simulink model "MyPTControl_RTW"  (R2022a)
settings: Solver=ode1  StartTime=0.0  StopTime=inf  FixedStep=0.001  RelTol=1e-3
PreLoadFcn:
  | vehicle = 'Car'; if ~length(which('cmself')), cmenv; end
  | MyPTControl_RTW_bus
InitFcn:
  | vehicle = 'Car'; if ~length(which('cmself')), cmenv; end
  | MyPTControl_RTW_bus
undefined symbols (not defined in the file or in its folder): EngineOut_Load, EngineOut_set_ISC, Ignition, ISGOut_Load, OperationState
libraries: simulink x11
(part 1 of 2)
Description:
  | CarMaker Plug-in Model Target
settings Model: ModifiedByFormat=IPG  Creator=ml  LastModifiedBy=IPG
settings DebuggingCC: UnconnectedInputMsg=warning  UnconnectedOutputMsg=warning  UnconnectedLineMsg=warning
settings RTWCC: Description=CarMaker Plug-in Model Target  SystemTargetFile=CarMaker.tlc  TemplateMakefile=CarMaker_unix-win64.tmf  DLArmComputeVersion=19.05
settings CodeAppCC: MaxIdLength=127
settings STFCustomTargetCC: TargetLangStandard=C99 (ISO)  CombineOutputUpdateFcns=on  MatFileLogging=on  CodeInterfacePackaging=Reusable function  GRTInterface=off  GenerateAllocFcn=on  SystemTargetFile=CarMaker.tlc
settings GRTTargetCC: ParMdlRefBuildCompliant=off  CompOptLevelCompliant=off  ConcurrentExecutionCompliant=off  CodeInterfacePackaging=Reusable function  CPPClassGenCompliant=off  GenerateAllocFcn=on  UseToolchainInfoCompliant=off

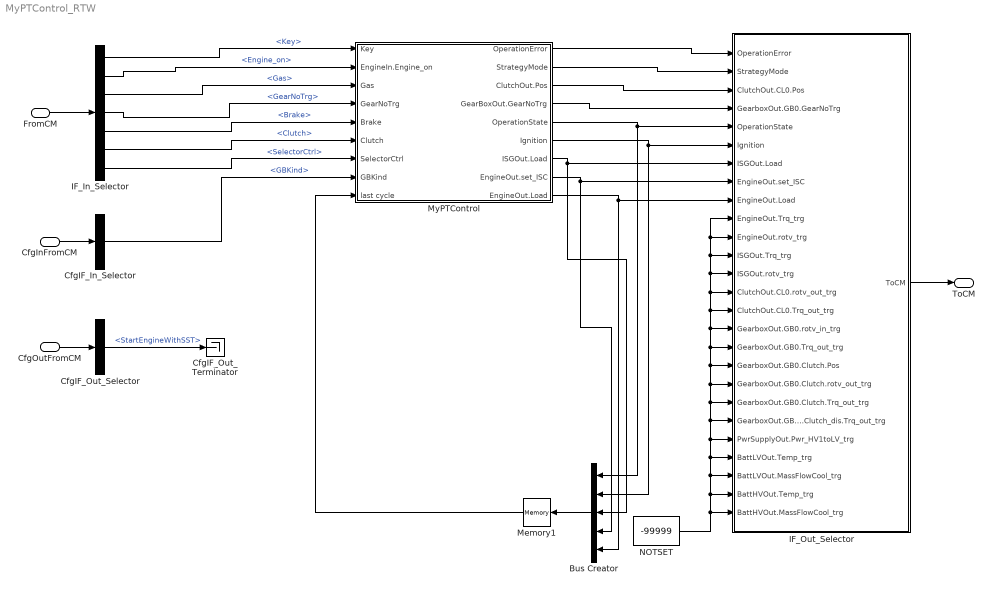
== system MyPTControl_RTW ==
  FromCM : Inport  OutDataTypeStr=Bus: cmPTControlIn
  CfgInFromCM : Inport  Port=2  OutDataTypeStr=Bus: cmPTControlCfgIn
  CfgOutFromCM : Inport  Port=3  OutDataTypeStr=Bus: cmPTControlCfgOut
  Bus Creator : BusCreator  Inputs=5
  CfgIF_In_Selector : BusSelector  OutputSignals=Gearbox.GB0.GBKind
  CfgIF_Out_Selector : BusSelector  OutputSignals=StartEngineWithSST
  CfgIF_Out_Terminator : Terminator
  IF_In_Selector : BusSelector  OutputSignals=Key,EngineIn.Engine_on,Gas,GearNoTrg,Brake,Clutch,SelectorCtrl
  IF_Out_Selector : Subsystem  mask(Signal Selection){}
      mask help: Signal Selection Block
      settings: OpenFcn=cmSignalSelect('SignalSelection_CB',gcb)
  Memory1 : Memory
  MyPTControl : Subsystem
  NOTSET : Constant  Value=-99999
  ToCM : Outport  OutDataTypeStr=Bus: cmPTControlOut
  wires:
  FromCM/1 -> IF_In_Selector/1
  IF_Out_Selector/1(ToCM) -> ToCM/1
  CfgInFromCM/1 -> CfgIF_In_Selector/1
  CfgOutFromCM/1 -> CfgIF_Out_Selector/1
  CfgIF_Out_Selector/1 -> CfgIF_Out_Terminator/1  "<StartEngineWithSST>"
  Bus Creator/1 -> Memory1/1
  MyPTControl/6(Ignition) -> IF_Out_Selector/6(Ignition), Bus Creator/2
  IF_In_Selector/2 -> MyPTControl/2(EngineIn.Engine_on)  "<Engine_on>"
  IF_In_Selector/6 -> MyPTControl/6(Clutch)  "<Clutch>"
  IF_In_Selector/3 -> MyPTControl/3(Gas)  "<Gas>"
  MyPTControl/1(OperationError) -> IF_Out_Selector/1(OperationError)
  CfgIF_In_Selector/1 -> MyPTControl/8(GBKind)  "<GBKind>"
  MyPTControl/4(GearBoxOut.GearNoTrg) -> IF_Out_Selector/4(GearboxOut.GB0.GearNoTrg)
  IF_In_Selector/4 -> MyPTControl/4(GearNoTrg)  "<GearNoTrg>"
  MyPTControl/7(ISGOut.Load) -> IF_Out_Selector/7(ISGOut.Load), Bus Creator/3
  IF_In_Selector/5 -> MyPTControl/5(Brake)  "<Brake>"
  MyPTControl/5(OperationState) -> IF_Out_Selector/5(OperationState), Bus Creator/1
  MyPTControl/8(EngineOut.set_ISC) -> IF_Out_Selector/8(EngineOut.set_ISC), Bus Creator/4
  IF_In_Selector/1 -> MyPTControl/1(Key)  "<Key>"
  MyPTControl/2(StrategyMode) -> IF_Out_Selector/2(StrategyMode)
  MyPTControl/3(ClutchOut.Pos) -> IF_Out_Selector/3(ClutchOut.CL0.Pos)
  Memory1/1 -> MyPTControl/9(last cycle)
  MyPTControl/9(EngineOut.Load) -> IF_Out_Selector/9(EngineOut.Load), Bus Creator/5
  NOTSET/1 -> IF_Out_Selector/26(BattHVOut.MassFlowCool_trg), IF_Out_Selector/25(BattHVOut.Temp_trg), IF_Out_Selector/24(BattLVOut.MassFlowCool_trg), IF_Out_Selector/23(BattLVOut.Temp_trg), IF_Out_Selector/22(PwrSupplyOut.Pwr_HV1toLV_trg), IF_Out_Selector/21(GearboxOut.GB0.Clutch_dis.Trq_out_trg), IF_Out_Selector/20(GearboxOut.GB0.Clutch.Trq_out_trg), IF_Out_Selector/19(GearboxOut.GB0.Clutch.rotv_out_trg), IF_Out_Selector/18(GearboxOut.GB0.Clutch.Pos), IF_Out_Selector/17(GearboxOut.GB0.Trq_out_trg), IF_Out_Selector/16(GearboxOut.GB0.rotv_in_trg), IF_Out_Selector/15(ClutchOut.CL0.Trq_out_trg), IF_Out_Selector/14(ClutchOut.CL0.rotv_out_trg), IF_Out_Selector/13(ISGOut.rotv_trg), IF_Out_Selector/12(ISGOut.Trq_trg), IF_Out_Selector/10(EngineOut.Trq_trg), IF_Out_Selector/11(EngineOut.rotv_trg)
  IF_In_Selector/7 -> MyPTControl/7(SelectorCtrl)  "<SelectorCtrl>"

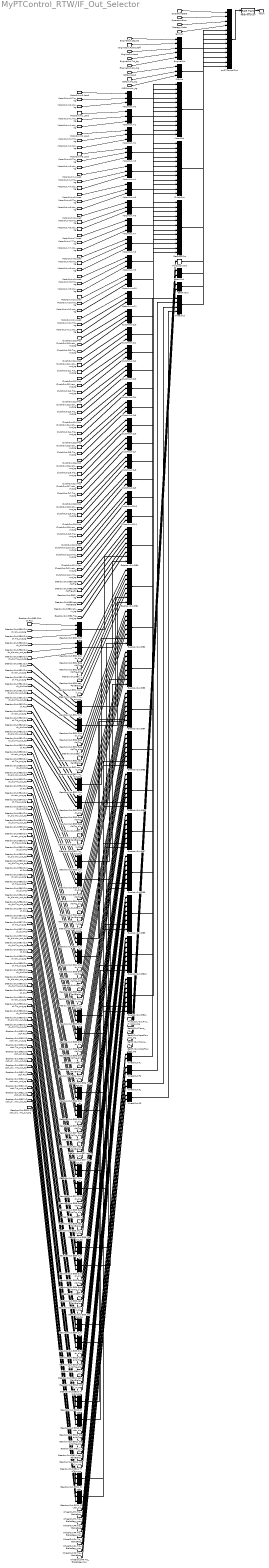
== system MyPTControl_RTW/IF_Out_Selector ==
  OperationError : Inport
  StrategyMode : Inport  Port=2
  ClutchOut.CL0.Pos : Inport  Port=3
  GearboxOut.GB0.GearNoTrg : Inport  Port=4
  OperationState : Inport  Port=5
  Ignition : Inport  Port=6
  ISGOut.Load : Inport  Port=7
  EngineOut.set_ISC : Inport  Port=8
  EngineOut.Load : Inport  Port=9
  EngineOut.Trq_trg : Inport  Port=10
  EngineOut.rotv_trg : Inport  Port=11
  ISGOut.Trq_trg : Inport  Port=12
  ISGOut.rotv_trg : Inport  Port=13
  ClutchOut.CL0.rotv_out_trg : Inport  Port=14
  ClutchOut.CL0.Trq_out_trg : Inport  Port=15
  GearboxOut.GB0.rotv_in_trg : Inport  Port=16
  GearboxOut.GB0.Trq_out_trg : Inport  Port=17
  GearboxOut.GB0.Clutch.Pos : Inport  Port=18
  GearboxOut.GB0.Clutch.rotv_out_trg : Inport  Port=19
  GearboxOut.GB0.Clutch.Trq_out_trg : Inport  Port=20
  GearboxOut.GB0.Clutch_dis.Trq_out_trg : Inport  Port=21
  PwrSupplyOut.Pwr_HV1toLV_trg : Inport  Port=22
  BattLVOut.Temp_trg : Inport  Port=23
  BattLVOut.MassFlowCool_trg : Inport  Port=24
  BattHVOut.Temp_trg : Inport  Port=25
  BattHVOut.MassFlowCool_trg : Inport  Port=26
  BattHVOut : BusCreator  Inputs=2
  BattLVOut : BusCreator  Inputs=2
  ClutchOut : BusCreator  Inputs=12
  ClutchOut.CL{0..11} (12 alike) : BusCreator  Inputs=3
  ClutchOut.CL1.Pos : Constant  Value=0
  ClutchOut.CL1.Trq_out_trg : Constant  Value=0
  ClutchOut.CL1.rotv_out_trg : Constant  Value=0
  ClutchOut.CL10.Pos : Constant  Value=0
  ClutchOut.CL10.Trq_out_trg : Constant  Value=0
  ClutchOut.CL10.rotv_out_trg : Constant  Value=0
  ClutchOut.CL11.Pos : Constant  Value=0
  ClutchOut.CL11.Trq_out_trg : Constant  Value=0
  ClutchOut.CL11.rotv_out_trg : Constant  Value=0
  ClutchOut.CL2.Pos : Constant  Value=0
  ClutchOut.CL2.Trq_out_trg : Constant  Value=0
  ClutchOut.CL2.rotv_out_trg : Constant  Value=0
  ClutchOut.CL3.Pos : Constant  Value=0
  ClutchOut.CL3.Trq_out_trg : Constant  Value=0
  ClutchOut.CL3.rotv_out_trg : Constant  Value=0
  ClutchOut.CL4.Pos : Constant  Value=0
  ClutchOut.CL4.Trq_out_trg : Constant  Value=0
  ClutchOut.CL4.rotv_out_trg : Constant  Value=0
  ClutchOut.CL5.Pos : Constant  Value=0
  ClutchOut.CL5.Trq_out_trg : Constant  Value=0
  ClutchOut.CL5.rotv_out_trg : Constant  Value=0
  ClutchOut.CL6.Pos : Constant  Value=0
  ClutchOut.CL6.Trq_out_trg : Constant  Value=0
  ClutchOut.CL6.rotv_out_trg : Constant  Value=0
  ClutchOut.CL7.Pos : Constant  Value=0
  ClutchOut.CL7.Trq_out_trg : Constant  Value=0
  ClutchOut.CL7.rotv_out_trg : Constant  Value=0
  ClutchOut.CL8.Pos : Constant  Value=0
  ClutchOut.CL8.Trq_out_trg : Constant  Value=0
  ClutchOut.CL8.rotv_out_trg : Constant  Value=0
  ClutchOut.CL9.Pos : Constant  Value=0
  ClutchOut.CL9.Trq_out_trg : Constant  Value=0
  ClutchOut.CL9.rotv_out_trg : Constant  Value=0
  EngineOut : BusCreator  Inputs=5
  EngineOut.FuelCutOff : Constant  Value=0
  GearboxOut : BusCreator  Inputs=12
  GearboxOut.GB{0..11} (12 alike) : BusCreator  Inputs=8
  GearboxOut.GB0.Clutch : BusCreator  Inputs=3
  GearboxOut.GB0.Clutch_dis : BusCreator  Inputs=3
  GearboxOut.GB0.Clutch_dis.Pos : Constant  Value=0
  GearboxOut.GB0.Clutch_dis.rotv_out_trg : Constant  Value=0
  GearboxOut.GB0.GearNoTrg_dis : Constant  Value=0
  GearboxOut.GB0.i_trg : Constant  Value=0
  GearboxOut.GB0.set_ParkBrake : Constant  Value=0
  GearboxOut.GB1.Clutch : BusCreator  Inputs=3
  GearboxOut.GB1.Clutch.Pos : Constant  Value=0
  GearboxOut.GB1.Clutch.Trq_out_trg : Constant  Value=0
  GearboxOut.GB1.Clutch.rotv_out_trg : Constant  Value=0
  GearboxOut.GB1.Clutch_dis : BusCreator  Inputs=3
  GearboxOut.GB1.Clutch_dis.Pos : Constant  Value=0
  GearboxOut.GB1.Clutch_dis.Trq_out_trg : Constant  Value=0
  GearboxOut.GB1.Clutch_dis.rotv_out_trg : Constant  Value=0
  GearboxOut.GB1.GearNoTrg : Constant  Value=0
  GearboxOut.GB1.GearNoTrg_dis : Constant  Value=0
  GearboxOut.GB1.Trq_out_trg : Constant  Value=0
  GearboxOut.GB1.i_trg : Constant  Value=0
  GearboxOut.GB1.rotv_in_trg : Constant  Value=0
  GearboxOut.GB1.set_ParkBrake : Constant  Value=0
  GearboxOut.GB10.Clutch : BusCreator  Inputs=3
  GearboxOut.GB10.Clutch.Pos : Constant  Value=0
  GearboxOut.GB10.Clutch.Trq_out_trg : Constant  Value=0
  GearboxOut.GB10.Clutch.rotv_out_trg : Constant  Value=0
  GearboxOut.GB10.Clutch_dis : BusCreator  Inputs=3
  GearboxOut.GB10.Clutch_dis.Pos : Constant  Value=0
  GearboxOut.GB10.Clutch_dis.Trq_out_trg : Constant  Value=0
  GearboxOut.GB10.Clutch_dis.rotv_out_trg : Constant  Value=0
  GearboxOut.GB10.GearNoTrg : Constant  Value=0
  GearboxOut.GB10.GearNoTrg_dis : Constant  Value=0
  GearboxOut.GB10.Trq_out_trg : Constant  Value=0
  GearboxOut.GB10.i_trg : Constant  Value=0
  GearboxOut.GB10.rotv_in_trg : Constant  Value=0
  GearboxOut.GB10.set_ParkBrake : Constant  Value=0
  GearboxOut.GB11.Clutch : BusCreator  Inputs=3
  GearboxOut.GB11.Clutch.Pos : Constant  Value=0
  GearboxOut.GB11.Clutch.Trq_out_trg : Constant  Value=0
  GearboxOut.GB11.Clutch.rotv_out_trg : Constant  Value=0
  GearboxOut.GB11.Clutch_dis : BusCreator  Inputs=3
  GearboxOut.GB11.Clutch_dis.Pos : Constant  Value=0
  GearboxOut.GB11.Clutch_dis.Trq_out_trg : Constant  Value=0
  GearboxOut.GB11.Clutch_dis.rotv_out_trg : Constant  Value=0
  GearboxOut.GB11.GearNoTrg : Constant  Value=0
  GearboxOut.GB11.GearNoTrg_dis : Constant  Value=0
  GearboxOut.GB11.Trq_out_trg : Constant  Value=0
  GearboxOut.GB11.i_trg : Constant  Value=0
  GearboxOut.GB11.rotv_in_trg : Constant  Value=0
  GearboxOut.GB11.set_ParkBrake : Constant  Value=0
  GearboxOut.GB2.Clutch : BusCreator  Inputs=3
  GearboxOut.GB2.Clutch.Pos : Constant  Value=0
  GearboxOut.GB2.Clutch.Trq_out_trg : Constant  Value=0
  GearboxOut.GB2.Clutch.rotv_out_trg : Constant  Value=0
  GearboxOut.GB2.Clutch_dis : BusCreator  Inputs=3
  GearboxOut.GB2.Clutch_dis.Pos : Constant  Value=0
  GearboxOut.GB2.Clutch_dis.Trq_out_trg : Constant  Value=0
  GearboxOut.GB2.Clutch_dis.rotv_out_trg : Constant  Value=0
  GearboxOut.GB2.GearNoTrg : Constant  Value=0
  GearboxOut.GB2.GearNoTrg_dis : Constant  Value=0
  GearboxOut.GB2.Trq_out_trg : Constant  Value=0
  GearboxOut.GB2.i_trg : Constant  Value=0
  GearboxOut.GB2.rotv_in_trg : Constant  Value=0
  GearboxOut.GB2.set_ParkBrake : Constant  Value=0
  GearboxOut.GB3.Clutch : BusCreator  Inputs=3
  GearboxOut.GB3.Clutch.Pos : Constant  Value=0
  GearboxOut.GB3.Clutch.Trq_out_trg : Constant  Value=0
  GearboxOut.GB3.Clutch.rotv_out_trg : Constant  Value=0
  GearboxOut.GB3.Clutch_dis : BusCreator  Inputs=3
  GearboxOut.GB3.Clutch_dis.Pos : Constant  Value=0
  GearboxOut.GB3.Clutch_dis.Trq_out_trg : Constant  Value=0
  GearboxOut.GB3.Clutch_dis.rotv_out_trg : Constant  Value=0
  GearboxOut.GB3.GearNoTrg : Constant  Value=0
  GearboxOut.GB3.GearNoTrg_dis : Constant  Value=0
  GearboxOut.GB3.Trq_out_trg : Constant  Value=0
  GearboxOut.GB3.i_trg : Constant  Value=0
  GearboxOut.GB3.rotv_in_trg : Constant  Value=0
  GearboxOut.GB3.set_ParkBrake : Constant  Value=0
  GearboxOut.GB4.Clutch : BusCreator  Inputs=3
  GearboxOut.GB4.Clutch.Pos : Constant  Value=0
  GearboxOut.GB4.Clutch.Trq_out_trg : Constant  Value=0
  GearboxOut.GB4.Clutch.rotv_out_trg : Constant  Value=0
  GearboxOut.GB4.Clutch_dis : BusCreator  Inputs=3
  GearboxOut.GB4.Clutch_dis.Pos : Constant  Value=0
  GearboxOut.GB4.Clutch_dis.Trq_out_trg : Constant  Value=0
  GearboxOut.GB4.Clutch_dis.rotv_out_trg : Constant  Value=0
  GearboxOut.GB4.GearNoTrg : Constant  Value=0
  GearboxOut.GB4.GearNoTrg_dis : Constant  Value=0
  GearboxOut.GB4.Trq_out_trg : Constant  Value=0
  GearboxOut.GB4.i_trg : Constant  Value=0
  GearboxOut.GB4.rotv_in_trg : Constant  Value=0
  GearboxOut.GB4.set_ParkBrake : Constant  Value=0
  GearboxOut.GB5.Clutch : BusCreator  Inputs=3
  GearboxOut.GB5.Clutch.Pos : Constant  Value=0
  GearboxOut.GB5.Clutch.Trq_out_trg : Constant  Value=0
  GearboxOut.GB5.Clutch.rotv_out_trg : Constant  Value=0
  GearboxOut.GB5.Clutch_dis : BusCreator  Inputs=3
  GearboxOut.GB5.Clutch_dis.Pos : Constant  Value=0
  GearboxOut.GB5.Clutch_dis.Trq_out_trg : Constant  Value=0
  GearboxOut.GB5.Clutch_dis.rotv_out_trg : Constant  Value=0
  GearboxOut.GB5.GearNoTrg : Constant  Value=0
  GearboxOut.GB5.GearNoTrg_dis : Constant  Value=0
  GearboxOut.GB5.Trq_out_trg : Constant  Value=0
  GearboxOut.GB5.i_trg : Constant  Value=0
  GearboxOut.GB5.rotv_in_trg : Constant  Value=0
  GearboxOut.GB5.set_ParkBrake : Constant  Value=0
  GearboxOut.GB6.Clutch : BusCreator  Inputs=3
  GearboxOut.GB6.Clutch.Pos : Constant  Value=0
  GearboxOut.GB6.Clutch.Trq_out_trg : Constant  Value=0
  GearboxOut.GB6.Clutch.rotv_out_trg : Constant  Value=0
  GearboxOut.GB6.Clutch_dis : BusCreator  Inputs=3
  GearboxOut.GB6.Clutch_dis.Pos : Constant  Value=0
  GearboxOut.GB6.Clutch_dis.Trq_out_trg : Constant  Value=0
  GearboxOut.GB6.Clutch_dis.rotv_out_trg : Constant  Value=0
  GearboxOut.GB6.GearNoTrg : Constant  Value=0
  GearboxOut.GB6.GearNoTrg_dis : Constant  Value=0
  GearboxOut.GB6.Trq_out_trg : Constant  Value=0
  GearboxOut.GB6.i_trg : Constant  Value=0
  GearboxOut.GB6.rotv_in_trg : Constant  Value=0
  GearboxOut.GB6.set_ParkBrake : Constant  Value=0
  GearboxOut.GB7.Clutch : BusCreator  Inputs=3
  GearboxOut.GB7.Clutch.Pos : Constant  Value=0
  GearboxOut.GB7.Clutch.Trq_out_trg : Constant  Value=0
  GearboxOut.GB7.Clutch.rotv_out_trg : Constant  Value=0
  GearboxOut.GB7.Clutch_dis : BusCreator  Inputs=3
  GearboxOut.GB7.Clutch_dis.Pos : Constant  Value=0
  GearboxOut.GB7.Clutch_dis.Trq_out_trg : Constant  Value=0
  GearboxOut.GB7.Clutch_dis.rotv_out_trg : Constant  Value=0
  GearboxOut.GB7.GearNoTrg : Constant  Value=0
  GearboxOut.GB7.GearNoTrg_dis : Constant  Value=0
  GearboxOut.GB7.Trq_out_trg : Constant  Value=0
  GearboxOut.GB7.i_trg : Constant  Value=0
  GearboxOut.GB7.rotv_in_trg : Constant  Value=0
  GearboxOut.GB7.set_ParkBrake : Constant  Value=0
  GearboxOut.GB8.Clutch : BusCreator  Inputs=3
  GearboxOut.GB8.Clutch.Pos : Constant  Value=0
  GearboxOut.GB8.Clutch.Trq_out_trg : Constant  Value=0
  GearboxOut.GB8.Clutch.rotv_out_trg : Constant  Value=0
  GearboxOut.GB8.Clutch_dis : BusCreator  Inputs=3
  GearboxOut.GB8.Clutch_dis.Pos : Constant  Value=0
  GearboxOut.GB8.Clutch_dis.Trq_out_trg : Constant  Value=0
  GearboxOut.GB8.Clutch_dis.rotv_out_trg : Constant  Value=0
  GearboxOut.GB8.GearNoTrg : Constant  Value=0
  GearboxOut.GB8.GearNoTrg_dis : Constant  Value=0
  GearboxOut.GB8.Trq_out_trg : Constant  Value=0
  GearboxOut.GB8.i_trg : Constant  Value=0
  GearboxOut.GB8.rotv_in_trg : Constant  Value=0
  GearboxOut.GB8.set_ParkBrake : Constant  Value=0
  GearboxOut.GB9.Clutch : BusCreator  Inputs=3
  GearboxOut.GB9.Clutch.Pos : Constant  Value=0
  GearboxOut.GB9.Clutch.Trq_out_trg : Constant  Value=0
  GearboxOut.GB9.Clutch.rotv_out_trg : Constant  Value=0
  GearboxOut.GB9.Clutch_dis : BusCreator  Inputs=3
  GearboxOut.GB9.Clutch_dis.Pos : Constant  Value=0
  GearboxOut.GB9.Clutch_dis.Trq_out_trg : Constant  Value=0
  GearboxOut.GB9.Clutch_dis.rotv_out_trg : Constant  Value=0
  GearboxOut.GB9.GearNoTrg : Constant  Value=0
  GearboxOut.GB9.GearNoTrg_dis : Constant  Value=0
  GearboxOut.GB9.Trq_out_trg : Constant  Value=0
  GearboxOut.GB9.i_trg : Constant  Value=0
  GearboxOut.GB9.rotv_in_trg : Constant  Value=0
  GearboxOut.GB9.set_ParkBrake : Constant  Value=0
  ISGOut : BusCreator  Inputs=3
  MotorOut : BusCreator  Inputs=12
  MotorOut.m{0..11} (12 alike) : BusCreator  Inputs=3
  MotorOut.m0.Load : Constant  Value=0
  MotorOut.m0.Trq_trg : Constant  Value=0
  MotorOut.m0.rotv_trg : Constant  Value=0
  MotorOut.m1.Load : Constant  Value=0
  MotorOut.m1.Trq_trg : Constant  Value=0
  MotorOut.m1.rotv_trg : Constant  Value=0
  MotorOut.m10.Load : Constant  Value=0
  MotorOut.m10.Trq_trg : Constant  Value=0
  MotorOut.m10.rotv_trg : Constant  Value=0
  MotorOut.m11.Load : Constant  Value=0
  MotorOut.m11.Trq_trg : Constant  Value=0
  MotorOut.m11.rotv_trg : Constant  Value=0
  MotorOut.m2.Load : Constant  Value=0
  MotorOut.m2.Trq_trg : Constant  Value=0
  MotorOut.m2.rotv_trg : Constant  Value=0
  MotorOut.m3.Load : Constant  Value=0
  MotorOut.m3.Trq_trg : Constant  Value=0
  MotorOut.m3.rotv_trg : Constant  Value=0
  MotorOut.m4.Load : Constant  Value=0
  MotorOut.m4.Trq_trg : Constant  Value=0
  MotorOut.m4.rotv_trg : Constant  Value=0
  MotorOut.m5.Load : Constant  Value=0
  MotorOut.m5.Trq_trg : Constant  Value=0
  MotorOut.m5.rotv_trg : Constant  Value=0
  MotorOut.m6.Load : Constant  Value=0
  MotorOut.m6.Trq_trg : Constant  Value=0
  MotorOut.m6.rotv_trg : Constant  Value=0
  MotorOut.m7.Load : Constant  Value=0
  MotorOut.m7.Trq_trg : Constant  Value=0
  MotorOut.m7.rotv_trg : Constant  Value=0
  MotorOut.m8.Load : Constant  Value=0
  MotorOut.m8.Trq_trg : Constant  Value=0
  MotorOut.m8.rotv_trg : Constant  Value=0
  MotorOut.m9.Load : Constant  Value=0
  MotorOut.m9.Trq_trg : Constant  Value=0
  MotorOut.m9.rotv_trg : Constant  Value=0
  PwrSupplyOut : BusCreator  Inputs=1
  RateTransition : RateTransition  OutPortSampleTime=str2num(get_param(bdroot,'FixedStep'))
  WheelOut : BusCreator  Inputs=4
  WheelOut.FL : BusCreator  Inputs=2
  WheelOut.FL.Trq_BrakeReg : Constant  Value=0
  WheelOut.FL.Trq_BrakeReg_max : Constant  Value=0
  WheelOut.FR : BusCreator  Inputs=2
  WheelOut.FR.Trq_BrakeReg : Constant  Value=0
  WheelOut.FR.Trq_BrakeReg_max : Constant  Value=0
  WheelOut.RL : BusCreator  Inputs=2
  WheelOut.RL.Trq_BrakeReg : Constant  Value=0
  WheelOut.RL.Trq_BrakeReg_max : Constant  Value=0
  WheelOut.RR : BusCreator  Inputs=2
  WheelOut.RR.Trq_BrakeReg : Constant  Value=0
  WheelOut.RR.Trq_BrakeReg_max : Constant  Value=0
  cmPTControlOut : BusCreator  Inputs=13
  ToCM : Outport
  wires:
  RateTransition/1 -> ToCM/1
  cmPTControlOut/1 -> RateTransition/1
  EngineOut/1 -> cmPTControlOut/5  "EngineOut"
  EngineOut.FuelCutOff/1 -> EngineOut/2  "FuelCutOff"
  ISGOut/1 -> cmPTControlOut/6  "ISGOut"
  MotorOut/1 -> cmPTControlOut/7  "MotorOut"
  MotorOut.m0/1 -> MotorOut/1  "m0"
  MotorOut.m0.Load/1 -> MotorOut.m0/1  "Load"
  MotorOut.m0.Trq_trg/1 -> MotorOut.m0/2  "Trq_trg"
  MotorOut.m0.rotv_trg/1 -> MotorOut.m0/3  "rotv_trg"
  MotorOut.m1/1 -> MotorOut/2  "m1"
  MotorOut.m1.Load/1 -> MotorOut.m1/1  "Load"
  MotorOut.m1.Trq_trg/1 -> MotorOut.m1/2  "Trq_trg"
  MotorOut.m1.rotv_trg/1 -> MotorOut.m1/3  "rotv_trg"
  MotorOut.m2/1 -> MotorOut/3  "m2"
  MotorOut.m2.Load/1 -> MotorOut.m2/1  "Load"
  MotorOut.m2.Trq_trg/1 -> MotorOut.m2/2  "Trq_trg"
  MotorOut.m2.rotv_trg/1 -> MotorOut.m2/3  "rotv_trg"
  MotorOut.m3/1 -> MotorOut/4  "m3"
  MotorOut.m3.Load/1 -> MotorOut.m3/1  "Load"
  MotorOut.m3.Trq_trg/1 -> MotorOut.m3/2  "Trq_trg"
  MotorOut.m3.rotv_trg/1 -> MotorOut.m3/3  "rotv_trg"
  MotorOut.m4/1 -> MotorOut/5  "m4"
  MotorOut.m4.Load/1 -> MotorOut.m4/1  "Load"
  MotorOut.m4.Trq_trg/1 -> MotorOut.m4/2  "Trq_trg"
  MotorOut.m4.rotv_trg/1 -> MotorOut.m4/3  "rotv_trg"
  MotorOut.m5/1 -> MotorOut/6  "m5"
  MotorOut.m5.Load/1 -> MotorOut.m5/1  "Load"
  MotorOut.m5.Trq_trg/1 -> MotorOut.m5/2  "Trq_trg"
  MotorOut.m5.rotv_trg/1 -> MotorOut.m5/3  "rotv_trg"
  MotorOut.m6/1 -> MotorOut/7  "m6"
  MotorOut.m6.Load/1 -> MotorOut.m6/1  "Load"
  MotorOut.m6.Trq_trg/1 -> MotorOut.m6/2  "Trq_trg"
  MotorOut.m6.rotv_trg/1 -> MotorOut.m6/3  "rotv_trg"
  MotorOut.m7/1 -> MotorOut/8  "m7"
  MotorOut.m7.Load/1 -> MotorOut.m7/1  "Load"
  MotorOut.m7.Trq_trg/1 -> MotorOut.m7/2  "Trq_trg"
  MotorOut.m7.rotv_trg/1 -> MotorOut.m7/3  "rotv_trg"
  MotorOut.m8/1 -> MotorOut/9  "m8"
  MotorOut.m8.Load/1 -> MotorOut.m8/1  "Load"
  MotorOut.m8.Trq_trg/1 -> MotorOut.m8/2  "Trq_trg"
  MotorOut.m8.rotv_trg/1 -> MotorOut.m8/3  "rotv_trg"
  MotorOut.m9/1 -> MotorOut/10  "m9"
  MotorOut.m9.Load/1 -> MotorOut.m9/1  "Load"
  MotorOut.m9.Trq_trg/1 -> MotorOut.m9/2  "Trq_trg"
  MotorOut.m9.rotv_trg/1 -> MotorOut.m9/3  "rotv_trg"
  MotorOut.m10/1 -> MotorOut/11  "m10"
  MotorOut.m10.Load/1 -> MotorOut.m10/1  "Load"
  MotorOut.m10.Trq_trg/1 -> MotorOut.m10/2  "Trq_trg"
  MotorOut.m10.rotv_trg/1 -> MotorOut.m10/3  "rotv_trg"
  MotorOut.m11/1 -> MotorOut/12  "m11"
  MotorOut.m11.Load/1 -> MotorOut.m11/1  "Load"
  MotorOut.m11.Trq_trg/1 -> MotorOut.m11/2  "Trq_trg"
  MotorOut.m11.rotv_trg/1 -> MotorOut.m11/3  "rotv_trg"
  ClutchOut/1 -> cmPTControlOut/8  "ClutchOut"
  ClutchOut.CL0/1 -> ClutchOut/1  "CL0"
  ClutchOut.CL1/1 -> ClutchOut/2  "CL1"
  ClutchOut.CL1.Pos/1 -> ClutchOut.CL1/1  "Pos"
  ClutchOut.CL1.rotv_out_trg/1 -> ClutchOut.CL1/2  "rotv_out_trg"
  ClutchOut.CL1.Trq_out_trg/1 -> ClutchOut.CL1/3  "Trq_out_trg"
  ClutchOut.CL2/1 -> ClutchOut/3  "CL2"
  ClutchOut.CL2.Pos/1 -> ClutchOut.CL2/1  "Pos"
  ClutchOut.CL2.rotv_out_trg/1 -> ClutchOut.CL2/2  "rotv_out_trg"
  ClutchOut.CL2.Trq_out_trg/1 -> ClutchOut.CL2/3  "Trq_out_trg"
  ClutchOut.CL3/1 -> ClutchOut/4  "CL3"
  ClutchOut.CL3.Pos/1 -> ClutchOut.CL3/1  "Pos"
  ClutchOut.CL3.rotv_out_trg/1 -> ClutchOut.CL3/2  "rotv_out_trg"
  ClutchOut.CL3.Trq_out_trg/1 -> ClutchOut.CL3/3  "Trq_out_trg"
  ClutchOut.CL4/1 -> ClutchOut/5  "CL4"
  ClutchOut.CL4.Pos/1 -> ClutchOut.CL4/1  "Pos"
  ClutchOut.CL4.rotv_out_trg/1 -> ClutchOut.CL4/2  "rotv_out_trg"
  ClutchOut.CL4.Trq_out_trg/1 -> ClutchOut.CL4/3  "Trq_out_trg"
  ClutchOut.CL5/1 -> ClutchOut/6  "CL5"
  ClutchOut.CL5.Pos/1 -> ClutchOut.CL5/1  "Pos"
  ClutchOut.CL5.rotv_out_trg/1 -> ClutchOut.CL5/2  "rotv_out_trg"
  ClutchOut.CL5.Trq_out_trg/1 -> ClutchOut.CL5/3  "Trq_out_trg"
  ClutchOut.CL6/1 -> ClutchOut/7  "CL6"
  ClutchOut.CL6.Pos/1 -> ClutchOut.CL6/1  "Pos"
  ClutchOut.CL6.rotv_out_trg/1 -> ClutchOut.CL6/2  "rotv_out_trg"
  ClutchOut.CL6.Trq_out_trg/1 -> ClutchOut.CL6/3  "Trq_out_trg"
  ClutchOut.CL7/1 -> ClutchOut/8  "CL7"
  ClutchOut.CL7.Pos/1 -> ClutchOut.CL7/1  "Pos"
  ClutchOut.CL7.rotv_out_trg/1 -> ClutchOut.CL7/2  "rotv_out_trg"
  ClutchOut.CL7.Trq_out_trg/1 -> ClutchOut.CL7/3  "Trq_out_trg"
  ClutchOut.CL8/1 -> ClutchOut/9  "CL8"
  ClutchOut.CL8.Pos/1 -> ClutchOut.CL8/1  "Pos"
  ClutchOut.CL8.rotv_out_trg/1 -> ClutchOut.CL8/2  "rotv_out_trg"
  ClutchOut.CL8.Trq_out_trg/1 -> ClutchOut.CL8/3  "Trq_out_trg"
  ClutchOut.CL9/1 -> ClutchOut/10  "CL9"
  ClutchOut.CL9.Pos/1 -> ClutchOut.CL9/1  "Pos"
  ClutchOut.CL9.rotv_out_trg/1 -> ClutchOut.CL9/2  "rotv_out_trg"
  ClutchOut.CL9.Trq_out_trg/1 -> ClutchOut.CL9/3  "Trq_out_trg"
  ClutchOut.CL10/1 -> ClutchOut/11  "CL10"
  ClutchOut.CL10.Pos/1 -> ClutchOut.CL10/1  "Pos"
  ClutchOut.CL10.rotv_out_trg/1 -> ClutchOut.CL10/2  "rotv_out_trg"
  ClutchOut.CL10.Trq_out_trg/1 -> ClutchOut.CL10/3  "Trq_out_trg"
  ClutchOut.CL11/1 -> ClutchOut/12  "CL11"
  ClutchOut.CL11.Pos/1 -> ClutchOut.CL11/1  "Pos"
  ClutchOut.CL11.rotv_out_trg/1 -> ClutchOut.CL11/2  "rotv_out_trg"
  ClutchOut.CL11.Trq_out_trg/1 -> ClutchOut.CL11/3  "Trq_out_trg"
  GearboxOut/1 -> cmPTControlOut/9  "GearboxOut"
  GearboxOut.GB0/1 -> GearboxOut/1  "GB0"
  GearboxOut.GB0.GearNoTrg_dis/1 -> GearboxOut.GB0/2  "GearNoTrg_dis"
  GearboxOut.GB0.i_trg/1 -> GearboxOut.GB0/3  "i_trg"
  GearboxOut.GB0.set_ParkBrake/1 -> GearboxOut.GB0/4  "set_ParkBrake"
  GearboxOut.GB0.Clutch/1 -> GearboxOut.GB0/7  "Clutch"
  GearboxOut.GB0.Clutch_dis/1 -> GearboxOut.GB0/8  "Clutch_dis"
  GearboxOut.GB0.Clutch_dis.Pos/1 -> GearboxOut.GB0.Clutch_dis/1  "Pos"
  GearboxOut.GB0.Clutch_dis.rotv_out_trg/1 -> GearboxOut.GB0.Clutch_dis/2  "rotv_out_trg"
  GearboxOut.GB1/1 -> GearboxOut/2  "GB1"
  GearboxOut.GB1.GearNoTrg/1 -> GearboxOut.GB1/1  "GearNoTrg"
  GearboxOut.GB1.GearNoTrg_dis/1 -> GearboxOut.GB1/2  "GearNoTrg_dis"
  GearboxOut.GB1.i_trg/1 -> GearboxOut.GB1/3  "i_trg"
  GearboxOut.GB1.set_ParkBrake/1 -> GearboxOut.GB1/4  "set_ParkBrake"
  GearboxOut.GB1.rotv_in_trg/1 -> GearboxOut.GB1/5  "rotv_in_trg"
  GearboxOut.GB1.Trq_out_trg/1 -> GearboxOut.GB1/6  "Trq_out_trg"
  GearboxOut.GB1.Clutch/1 -> GearboxOut.GB1/7  "Clutch"
  GearboxOut.GB1.Clutch.Pos/1 -> GearboxOut.GB1.Clutch/1  "Pos"
  GearboxOut.GB1.Clutch.rotv_out_trg/1 -> GearboxOut.GB1.Clutch/2  "rotv_out_trg"
  GearboxOut.GB1.Clutch.Trq_out_trg/1 -> GearboxOut.GB1.Clutch/3  "Trq_out_trg"
  GearboxOut.GB1.Clutch_dis/1 -> GearboxOut.GB1/8  "Clutch_dis"
  GearboxOut.GB1.Clutch_dis.Pos/1 -> GearboxOut.GB1.Clutch_dis/1  "Pos"
  GearboxOut.GB1.Clutch_dis.rotv_out_trg/1 -> GearboxOut.GB1.Clutch_dis/2  "rotv_out_trg"
  GearboxOut.GB1.Clutch_dis.Trq_out_trg/1 -> GearboxOut.GB1.Clutch_dis/3  "Trq_out_trg"
  GearboxOut.GB2/1 -> GearboxOut/3  "GB2"
  GearboxOut.GB2.GearNoTrg/1 -> GearboxOut.GB2/1  "GearNoTrg"
  GearboxOut.GB2.GearNoTrg_dis/1 -> GearboxOut.GB2/2  "GearNoTrg_dis"
  GearboxOut.GB2.i_trg/1 -> GearboxOut.GB2/3  "i_trg"
  GearboxOut.GB2.set_ParkBrake/1 -> GearboxOut.GB2/4  "set_ParkBrake"
  GearboxOut.GB2.rotv_in_trg/1 -> GearboxOut.GB2/5  "rotv_in_trg"
  GearboxOut.GB2.Trq_out_trg/1 -> GearboxOut.GB2/6  "Trq_out_trg"
  GearboxOut.GB2.Clutch/1 -> GearboxOut.GB2/7  "Clutch"
  GearboxOut.GB2.Clutch.Pos/1 -> GearboxOut.GB2.Clutch/1  "Pos"
  GearboxOut.GB2.Clutch.rotv_out_trg/1 -> GearboxOut.GB2.Clutch/2  "rotv_out_trg"
  GearboxOut.GB2.Clutch.Trq_out_trg/1 -> GearboxOut.GB2.Clutch/3  "Trq_out_trg"
  GearboxOut.GB2.Clutch_dis/1 -> GearboxOut.GB2/8  "Clutch_dis"
  GearboxOut.GB2.Clutch_dis.Pos/1 -> GearboxOut.GB2.Clutch_dis/1  "Pos"
  GearboxOut.GB2.Clutch_dis.rotv_out_trg/1 -> GearboxOut.GB2.Clutch_dis/2  "rotv_out_trg"
  GearboxOut.GB2.Clutch_dis.Trq_out_trg/1 -> GearboxOut.GB2.Clutch_dis/3  "Trq_out_trg"
  GearboxOut.GB3/1 -> GearboxOut/4  "GB3"
  GearboxOut.GB3.GearNoTrg/1 -> GearboxOut.GB3/1  "GearNoTrg"
  GearboxOut.GB3.GearNoTrg_dis/1 -> GearboxOut.GB3/2  "GearNoTrg_dis"
  GearboxOut.GB3.i_trg/1 -> GearboxOut.GB3/3  "i_trg"
  GearboxOut.GB3.set_ParkBrake/1 -> GearboxOut.GB3/4  "set_ParkBrake"
  GearboxOut.GB3.rotv_in_trg/1 -> GearboxOut.GB3/5  "rotv_in_trg"
  GearboxOut.GB3.Trq_out_trg/1 -> GearboxOut.GB3/6  "Trq_out_trg"
  GearboxOut.GB3.Clutch/1 -> GearboxOut.GB3/7  "Clutch"
  GearboxOut.GB3.Clutch.Pos/1 -> GearboxOut.GB3.Clutch/1  "Pos"
  GearboxOut.GB3.Clutch.rotv_out_trg/1 -> GearboxOut.GB3.Clutch/2  "rotv_out_trg"
  GearboxOut.GB3.Clutch.Trq_out_trg/1 -> GearboxOut.GB3.Clutch/3  "Trq_out_trg"
  GearboxOut.GB3.Clutch_dis/1 -> GearboxOut.GB3/8  "Clutch_dis"
  GearboxOut.GB3.Clutch_dis.Pos/1 -> GearboxOut.GB3.Clutch_dis/1  "Pos"
  GearboxOut.GB3.Clutch_dis.rotv_out_trg/1 -> GearboxOut.GB3.Clutch_dis/2  "rotv_out_trg"
  GearboxOut.GB3.Clutch_dis.Trq_out_trg/1 -> GearboxOut.GB3.Clutch_dis/3  "Trq_out_trg"
  GearboxOut.GB4/1 -> GearboxOut/5  "GB4"
  GearboxOut.GB4.GearNoTrg/1 -> GearboxOut.GB4/1  "GearNoTrg"
  GearboxOut.GB4.GearNoTrg_dis/1 -> GearboxOut.GB4/2  "GearNoTrg_dis"
  GearboxOut.GB4.i_trg/1 -> GearboxOut.GB4/3  "i_trg"
  GearboxOut.GB4.set_ParkBrake/1 -> GearboxOut.GB4/4  "set_ParkBrake"
  GearboxOut.GB4.rotv_in_trg/1 -> GearboxOut.GB4/5  "rotv_in_trg"
  GearboxOut.GB4.Trq_out_trg/1 -> GearboxOut.GB4/6  "Trq_out_trg"
  GearboxOut.GB4.Clutch/1 -> GearboxOut.GB4/7  "Clutch"
  GearboxOut.GB4.Clutch.Pos/1 -> GearboxOut.GB4.Clutch/1  "Pos"
  GearboxOut.GB4.Clutch.rotv_out_trg/1 -> GearboxOut.GB4.Clutch/2  "rotv_out_trg"
  GearboxOut.GB4.Clutch.Trq_out_trg/1 -> GearboxOut.GB4.Clutch/3  "Trq_out_trg"
  GearboxOut.GB4.Clutch_dis/1 -> GearboxOut.GB4/8  "Clutch_dis"
  GearboxOut.GB4.Clutch_dis.Pos/1 -> GearboxOut.GB4.Clutch_dis/1  "Pos"
  GearboxOut.GB4.Clutch_dis.rotv_out_trg/1 -> GearboxOut.GB4.Clutch_dis/2  "rotv_out_trg"
  GearboxOut.GB4.Clutch_dis.Trq_out_trg/1 -> GearboxOut.GB4.Clutch_dis/3  "Trq_out_trg"
  GearboxOut.GB5/1 -> GearboxOut/6  "GB5"
  GearboxOut.GB5.GearNoTrg/1 -> GearboxOut.GB5/1  "GearNoTrg"
  GearboxOut.GB5.GearNoTrg_dis/1 -> GearboxOut.GB5/2  "GearNoTrg_dis"
  GearboxOut.GB5.i_trg/1 -> GearboxOut.GB5/3  "i_trg"
  GearboxOut.GB5.set_ParkBrake/1 -> GearboxOut.GB5/4  "set_ParkBrake"
  GearboxOut.GB5.rotv_in_trg/1 -> GearboxOut.GB5/5  "rotv_in_trg"
  GearboxOut.GB5.Trq_out_trg/1 -> GearboxOut.GB5/6  "Trq_out_trg"
  GearboxOut.GB5.Clutch/1 -> GearboxOut.GB5/7  "Clutch"
  GearboxOut.GB5.Clutch.Pos/1 -> GearboxOut.GB5.Clutch/1  "Pos"
  GearboxOut.GB5.Clutch.rotv_out_trg/1 -> GearboxOut.GB5.Clutch/2  "rotv_out_trg"
  GearboxOut.GB5.Clutch.Trq_out_trg/1 -> GearboxOut.GB5.Clutch/3  "Trq_out_trg"
  GearboxOut.GB5.Clutch_dis/1 -> GearboxOut.GB5/8  "Clutch_dis"
  GearboxOut.GB5.Clutch_dis.Pos/1 -> GearboxOut.GB5.Clutch_dis/1  "Pos"
  GearboxOut.GB5.Clutch_dis.rotv_out_trg/1 -> GearboxOut.GB5.Clutch_dis/2  "rotv_out_trg"
  GearboxOut.GB5.Clutch_dis.Trq_out_trg/1 -> GearboxOut.GB5.Clutch_dis/3  "Trq_out_trg"
  GearboxOut.GB6/1 -> GearboxOut/7  "GB6"
  GearboxOut.GB6.GearNoTrg/1 -> GearboxOut.GB6/1  "GearNoTrg"
  GearboxOut.GB6.GearNoTrg_dis/1 -> GearboxOut.GB6/2  "GearNoTrg_dis"
  GearboxOut.GB6.i_trg/1 -> GearboxOut.GB6/3  "i_trg"
  GearboxOut.GB6.set_ParkBrake/1 -> GearboxOut.GB6/4  "set_ParkBrake"
  GearboxOut.GB6.rotv_in_trg/1 -> GearboxOut.GB6/5  "rotv_in_trg"
  GearboxOut.GB6.Trq_out_trg/1 -> GearboxOut.GB6/6  "Trq_out_trg"
  GearboxOut.GB6.Clutch/1 -> GearboxOut.GB6/7  "Clutch"
  GearboxOut.GB6.Clutch.Pos/1 -> GearboxOut.GB6.Clutch/1  "Pos"
  GearboxOut.GB6.Clutch.rotv_out_trg/1 -> GearboxOut.GB6.Clutch/2  "rotv_out_trg"
  GearboxOut.GB6.Clutch.Trq_out_trg/1 -> GearboxOut.GB6.Clutch/3  "Trq_out_trg"
  GearboxOut.GB6.Clutch_dis/1 -> GearboxOut.GB6/8  "Clutch_dis"
  GearboxOut.GB6.Clutch_dis.Pos/1 -> GearboxOut.GB6.Clutch_dis/1  "Pos"
  GearboxOut.GB6.Clutch_dis.rotv_out_trg/1 -> GearboxOut.GB6.Clutch_dis/2  "rotv_out_trg"
  GearboxOut.GB6.Clutch_dis.Trq_out_trg/1 -> GearboxOut.GB6.Clutch_dis/3  "Trq_out_trg"
  GearboxOut.GB7/1 -> GearboxOut/8  "GB7"
  GearboxOut.GB7.GearNoTrg/1 -> GearboxOut.GB7/1  "GearNoTrg"
  GearboxOut.GB7.GearNoTrg_dis/1 -> GearboxOut.GB7/2  "GearNoTrg_dis"
  GearboxOut.GB7.i_trg/1 -> GearboxOut.GB7/3  "i_trg"
  GearboxOut.GB7.set_ParkBrake/1 -> GearboxOut.GB7/4  "set_ParkBrake"
  GearboxOut.GB7.rotv_in_trg/1 -> GearboxOut.GB7/5  "rotv_in_trg"
  GearboxOut.GB7.Trq_out_trg/1 -> GearboxOut.GB7/6  "Trq_out_trg"
  GearboxOut.GB7.Clutch/1 -> GearboxOut.GB7/7  "Clutch"
  GearboxOut.GB7.Clutch.Pos/1 -> GearboxOut.GB7.Clutch/1  "Pos"
  GearboxOut.GB7.Clutch.rotv_out_trg/1 -> GearboxOut.GB7.Clutch/2  "rotv_out_trg"
  GearboxOut.GB7.Clutch.Trq_out_trg/1 -> GearboxOut.GB7.Clutch/3  "Trq_out_trg"
  GearboxOut.GB7.Clutch_dis/1 -> GearboxOut.GB7/8  "Clutch_dis"
  GearboxOut.GB7.Clutch_dis.Pos/1 -> GearboxOut.GB7.Clutch_dis/1  "Pos"
  GearboxOut.GB7.Clutch_dis.rotv_out_trg/1 -> GearboxOut.GB7.Clutch_dis/2  "rotv_out_trg"
  GearboxOut.GB7.Clutch_dis.Trq_out_trg/1 -> GearboxOut.GB7.Clutch_dis/3  "Trq_out_trg"
  GearboxOut.GB8/1 -> GearboxOut/9  "GB8"
  GearboxOut.GB8.GearNoTrg/1 -> GearboxOut.GB8/1  "GearNoTrg"
  GearboxOut.GB8.GearNoTrg_dis/1 -> GearboxOut.GB8/2  "GearNoTrg_dis"
  GearboxOut.GB8.i_trg/1 -> GearboxOut.GB8/3  "i_trg"
  GearboxOut.GB8.set_ParkBrake/1 -> GearboxOut.GB8/4  "set_ParkBrake"
  GearboxOut.GB8.rotv_in_trg/1 -> GearboxOut.GB8/5  "rotv_in_trg"
  GearboxOut.GB8.Trq_out_trg/1 -> GearboxOut.GB8/6  "Trq_out_trg"
  GearboxOut.GB8.Clutch/1 -> GearboxOut.GB8/7  "Clutch"
  GearboxOut.GB8.Clutch.Pos/1 -> GearboxOut.GB8.Clutch/1  "Pos"
  GearboxOut.GB8.Clutch.rotv_out_trg/1 -> GearboxOut.GB8.Clutch/2  "rotv_out_trg"
  GearboxOut.GB8.Clutch.Trq_out_trg/1 -> GearboxOut.GB8.Clutch/3  "Trq_out_trg"
  GearboxOut.GB8.Clutch_dis/1 -> GearboxOut.GB8/8  "Clutch_dis"
  GearboxOut.GB8.Clutch_dis.Pos/1 -> GearboxOut.GB8.Clutch_dis/1  "Pos"
  GearboxOut.GB8.Clutch_dis.rotv_out_trg/1 -> GearboxOut.GB8.Clutch_dis/2  "rotv_out_trg"
  GearboxOut.GB8.Clutch_dis.Trq_out_trg/1 -> GearboxOut.GB8.Clutch_dis/3  "Trq_out_trg"
  GearboxOut.GB9/1 -> GearboxOut/10  "GB9"
  GearboxOut.GB9.GearNoTrg/1 -> GearboxOut.GB9/1  "GearNoTrg"
  GearboxOut.GB9.GearNoTrg_dis/1 -> GearboxOut.GB9/2  "GearNoTrg_dis"
  GearboxOut.GB9.i_trg/1 -> GearboxOut.GB9/3  "i_trg"
  GearboxOut.GB9.set_ParkBrake/1 -> GearboxOut.GB9/4  "set_ParkBrake"
  GearboxOut.GB9.rotv_in_trg/1 -> GearboxOut.GB9/5  "rotv_in_trg"
  GearboxOut.GB9.Trq_out_trg/1 -> GearboxOut.GB9/6  "Trq_out_trg"
  GearboxOut.GB9.Clutch/1 -> GearboxOut.GB9/7  "Clutch"
  GearboxOut.GB9.Clutch.Pos/1 -> GearboxOut.GB9.Clutch/1  "Pos"
  GearboxOut.GB9.Clutch.rotv_out_trg/1 -> GearboxOut.GB9.Clutch/2  "rotv_out_trg"
  GearboxOut.GB9.Clutch.Trq_out_trg/1 -> GearboxOut.GB9.Clutch/3  "Trq_out_trg"
  GearboxOut.GB9.Clutch_dis/1 -> GearboxOut.GB9/8  "Clutch_dis"
  GearboxOut.GB9.Clutch_dis.Pos/1 -> GearboxOut.GB9.Clutch_dis/1  "Pos"
  GearboxOut.GB9.Clutch_dis.rotv_out_trg/1 -> GearboxOut.GB9.Clutch_dis/2  "rotv_out_trg"
  GearboxOut.GB9.Clutch_dis.Trq_out_trg/1 -> GearboxOut.GB9.Clutch_dis/3  "Trq_out_trg"
  GearboxOut.GB10/1 -> GearboxOut/11  "GB10"
  GearboxOut.GB10.GearNoTrg/1 -> GearboxOut.GB10/1  "GearNoTrg"
  GearboxOut.GB10.GearNoTrg_dis/1 -> GearboxOut.GB10/2  "GearNoTrg_dis"
  GearboxOut.GB10.i_trg/1 -> GearboxOut.GB10/3  "i_trg"
  GearboxOut.GB10.set_ParkBrake/1 -> GearboxOut.GB10/4  "set_ParkBrake"
  GearboxOut.GB10.rotv_in_trg/1 -> GearboxOut.GB10/5  "rotv_in_trg"
  GearboxOut.GB10.Trq_out_trg/1 -> GearboxOut.GB10/6  "Trq_out_trg"
  GearboxOut.GB10.Clutch/1 -> GearboxOut.GB10/7  "Clutch"
  GearboxOut.GB10.Clutch.Pos/1 -> GearboxOut.GB10.Clutch/1  "Pos"
  GearboxOut.GB10.Clutch.rotv_out_trg/1 -> GearboxOut.GB10.Clutch/2  "rotv_out_trg"
  GearboxOut.GB10.Clutch.Trq_out_trg/1 -> GearboxOut.GB10.Clutch/3  "Trq_out_trg"
  GearboxOut.GB10.Clutch_dis/1 -> GearboxOut.GB10/8  "Clutch_dis"
  GearboxOut.GB10.Clutch_dis.Pos/1 -> GearboxOut.GB10.Clutch_dis/1  "Pos"
  GearboxOut.GB10.Clutch_dis.rotv_out_trg/1 -> GearboxOut.GB10.Clutch_dis/2  "rotv_out_trg"
  GearboxOut.GB10.Clutch_dis.Trq_out_trg/1 -> GearboxOut.GB10.Clutch_dis/3  "Trq_out_trg"
  GearboxOut.GB11/1 -> GearboxOut/12  "GB11"
  GearboxOut.GB11.GearNoTrg/1 -> GearboxOut.GB11/1  "GearNoTrg"
  GearboxOut.GB11.GearNoTrg_dis/1 -> GearboxOut.GB11/2  "GearNoTrg_dis"
  GearboxOut.GB11.i_trg/1 -> GearboxOut.GB11/3  "i_trg"
  GearboxOut.GB11.set_ParkBrake/1 -> GearboxOut.GB11/4  "set_ParkBrake"
  GearboxOut.GB11.rotv_in_trg/1 -> GearboxOut.GB11/5  "rotv_in_trg"
  GearboxOut.GB11.Trq_out_trg/1 -> GearboxOut.GB11/6  "Trq_out_trg"
  GearboxOut.GB11.Clutch/1 -> GearboxOut.GB11/7  "Clutch"
  GearboxOut.GB11.Clutch.Pos/1 -> GearboxOut.GB11.Clutch/1  "Pos"
  GearboxOut.GB11.Clutch.rotv_out_trg/1 -> GearboxOut.GB11.Clutch/2  "rotv_out_trg"
  GearboxOut.GB11.Clutch.Trq_out_trg/1 -> GearboxOut.GB11.Clutch/3  "Trq_out_trg"
  GearboxOut.GB11.Clutch_dis/1 -> GearboxOut.GB11/8  "Clutch_dis"
  GearboxOut.GB11.Clutch_dis.Pos/1 -> GearboxOut.GB11.Clutch_dis/1  "Pos"
  GearboxOut.GB11.Clutch_dis.rotv_out_trg/1 -> GearboxOut.GB11.Clutch_dis/2  "rotv_out_trg"
  GearboxOut.GB11.Clutch_dis.Trq_out_trg/1 -> GearboxOut.GB11.Clutch_dis/3  "Trq_out_trg"
  PwrSupplyOut/1 -> cmPTControlOut/10  "PwrSupplyOut"
  BattLVOut/1 -> cmPTControlOut/11  "BattLVOut"
  BattHVOut/1 -> cmPTControlOut/12  "BattHVOut"
  WheelOut/1 -> cmPTControlOut/13  "WheelOut"
  WheelOut.FL/1 -> WheelOut/1  "FL"
  WheelOut.FL.Trq_BrakeReg/1 -> WheelOut.FL/1  "Trq_BrakeReg"
  WheelOut.FL.Trq_BrakeReg_max/1 -> WheelOut.FL/2  "Trq_BrakeReg_max"
  WheelOut.FR/1 -> WheelOut/2  "FR"
  WheelOut.FR.Trq_BrakeReg/1 -> WheelOut.FR/1  "Trq_BrakeReg"
  WheelOut.FR.Trq_BrakeReg_max/1 -> WheelOut.FR/2  "Trq_BrakeReg_max"
  WheelOut.RL/1 -> WheelOut/3  "RL"
  WheelOut.RL.Trq_BrakeReg/1 -> WheelOut.RL/1  "Trq_BrakeReg"
  WheelOut.RL.Trq_BrakeReg_max/1 -> WheelOut.RL/2  "Trq_BrakeReg_max"
  WheelOut.RR/1 -> WheelOut/4  "RR"
  WheelOut.RR.Trq_BrakeReg/1 -> WheelOut.RR/1  "Trq_BrakeReg"
  WheelOut.RR.Trq_BrakeReg_max/1 -> WheelOut.RR/2  "Trq_BrakeReg_max"
  OperationError/1 -> cmPTControlOut/2  "OperationError"
  StrategyMode/1 -> cmPTControlOut/3  "StrategyMode"
  ClutchOut.CL0.Pos/1 -> ClutchOut.CL0/1  "Pos"
  GearboxOut.GB0.GearNoTrg/1 -> GearboxOut.GB0/1  "GearNoTrg"
  OperationState/1 -> cmPTControlOut/1  "OperationState"
  Ignition/1 -> cmPTControlOut/4  "Ignition"
  ISGOut.Load/1 -> ISGOut/1  "Load"
  EngineOut.set_ISC/1 -> EngineOut/1  "set_ISC"
  EngineOut.Load/1 -> EngineOut/3  "Load"
  EngineOut.Trq_trg/1 -> EngineOut/4  "Trq_trg"
  EngineOut.rotv_trg/1 -> EngineOut/5  "rotv_trg"
  ISGOut.Trq_trg/1 -> ISGOut/2  "Trq_trg"
  ISGOut.rotv_trg/1 -> ISGOut/3  "rotv_trg"
  ClutchOut.CL0.rotv_out_trg/1 -> ClutchOut.CL0/2  "rotv_out_trg"
  ClutchOut.CL0.Trq_out_trg/1 -> ClutchOut.CL0/3  "Trq_out_trg"
  GearboxOut.GB0.rotv_in_trg/1 -> GearboxOut.GB0/5  "rotv_in_trg"
  GearboxOut.GB0.Trq_out_trg/1 -> GearboxOut.GB0/6  "Trq_out_trg"
  GearboxOut.GB0.Clutch.Pos/1 -> GearboxOut.GB0.Clutch/1  "Pos"
  GearboxOut.GB0.Clutch.rotv_out_trg/1 -> GearboxOut.GB0.Clutch/2  "rotv_out_trg"
  GearboxOut.GB0.Clutch.Trq_out_trg/1 -> GearboxOut.GB0.Clutch/3  "Trq_out_trg"
  GearboxOut.GB0.Clutch_dis.Trq_out_trg/1 -> GearboxOut.GB0.Clutch_dis/3  "Trq_out_trg"
  PwrSupplyOut.Pwr_HV1toLV_trg/1 -> PwrSupplyOut/1  "Pwr_HV1toLV_trg"
  BattLVOut.Temp_trg/1 -> BattLVOut/1  "Temp_trg"
  BattLVOut.MassFlowCool_trg/1 -> BattLVOut/2  "MassFlowCool_trg"
  BattHVOut.Temp_trg/1 -> BattHVOut/1  "Temp_trg"
  BattHVOut.MassFlowCool_trg/1 -> BattHVOut/2  "MassFlowCool_trg"

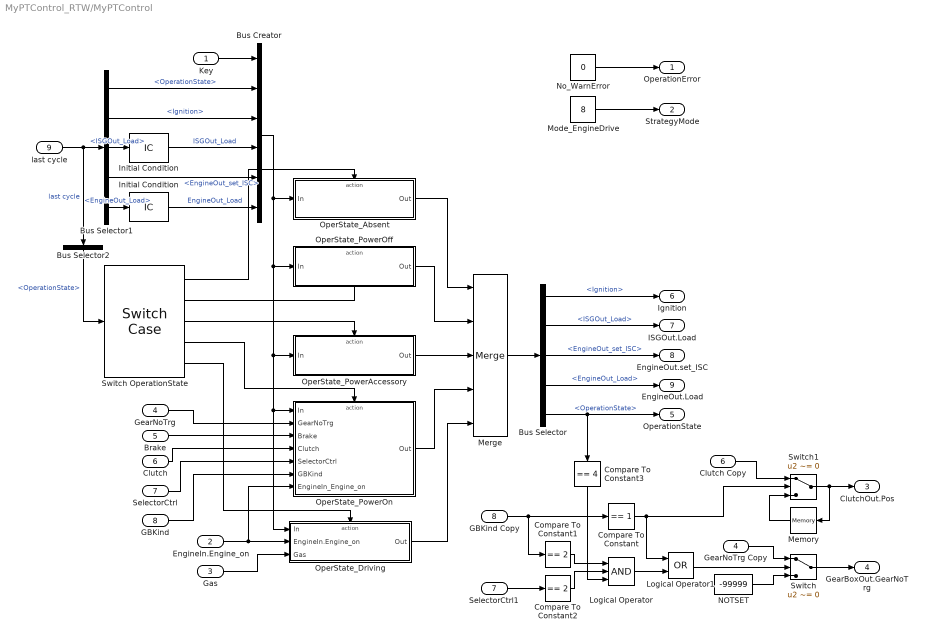
== system MyPTControl_RTW/MyPTControl ==
  Key : Inport
  EngineIn.Engine_on : Inport  Port=2
  Gas : Inport  Port=3
  GearNoTrg : Inport  Port=4
  Brake : Inport  Port=5
  Clutch : Inport  Port=6
  SelectorCtrl : Inport  Port=7
  GBKind : Inport  Port=8
  last cycle : Inport  Port=9
  Bus Creator : BusCreator  Inputs=6
  Bus Selector : BusSelector  OutputSignals=Ignition,ISGOut_Load,EngineOut_set_ISC,EngineOut_Load,OperationState
  Bus Selector1 : BusSelector  OutputSignals=OperationState,Ignition,ISGOut_Load,EngineOut_set_ISC,EngineOut_Load
  Bus Selector2 : BusSelector  OutputSignals=OperationState
  Clutch Copy : InportShadow  Port=6
  Compare To Constant : simulink/Logic and Bit Operations/Compare To Constant  relop===  const=1  OutDataTypeStr=uint8  ZeroCross=off
  Compare To Constant1 : simulink/Logic and Bit Operations/Compare To Constant  relop===  const=2  OutDataTypeStr=uint8  ZeroCross=off
  Compare To Constant2 : simulink/Logic and Bit Operations/Compare To Constant  relop===  const=2  OutDataTypeStr=uint8  ZeroCross=off
  Compare To Constant3 : simulink/Logic and Bit Operations/Compare To Constant  relop===  const=4  OutDataTypeStr=uint8  ZeroCross=off
  GBKind Copy : InportShadow  Port=8
  GearNoTrg Copy : InportShadow  Port=4
  Initial Condition : InitialCondition  Value=0
  "Initial Condition " : InitialCondition  Value=0
  Logical Operator : Logic  Inputs=3  AllPortsSameDT=off  OutDataTypeStr=boolean
  Logical Operator1 : Logic  Operator=OR  AllPortsSameDT=off  OutDataTypeStr=boolean
  Memory : Memory
  Merge : Merge  Inputs=5
  Mode_EngineDrive : Constant  Value=8
  NOTSET : Constant  Value=-99999
  No_WarnError : Constant  Value=0
  OperState_Absent : Subsystem  TreatAsAtomicUnit=on
  OperState_Driving : Subsystem  TreatAsAtomicUnit=on
  OperState_PowerAccessory : Subsystem  TreatAsAtomicUnit=on
  OperState_PowerOff : Subsystem  TreatAsAtomicUnit=on
  OperState_PowerOn : Subsystem  TreatAsAtomicUnit=on
  SelectorCtrl1 : InportShadow  Port=7
  Switch : Switch  Criteria=u2 ~= 0  SaturateOnIntegerOverflow=off  InputSameDT=off
  Switch OperationState : SwitchCase  CaseConditions={0 1 2 3}
  Switch1 : Switch  Criteria=u2 ~= 0  SaturateOnIntegerOverflow=off  InputSameDT=off
  OperationError : Outport  VectorParamsAs1DForOutWhenUnconnected=off
  StrategyMode : Outport  Port=2  VectorParamsAs1DForOutWhenUnconnected=off
  ClutchOut.Pos : Outport  Port=3  VectorParamsAs1DForOutWhenUnconnected=off
  GearBoxOut.GearNoTrg : Outport  Port=4  VectorParamsAs1DForOutWhenUnconnected=off
  OperationState : Outport  Port=5  VectorParamsAs1DForOutWhenUnconnected=off
  Ignition : Outport  Port=6  VectorParamsAs1DForOutWhenUnconnected=off
  ISGOut.Load : Outport  Port=7  VectorParamsAs1DForOutWhenUnconnected=off
  EngineOut.set_ISC : Outport  Port=8  VectorParamsAs1DForOutWhenUnconnected=off
  EngineOut.Load : Outport  Port=9  VectorParamsAs1DForOutWhenUnconnected=off
  wires:
  Compare To Constant3/1 -> Logical Operator/3
  GBKind Copy/1 -> Compare To Constant1/1, Compare To Constant/1
  SelectorCtrl1/1 -> Compare To Constant2/1
  OperState_Absent/1(Out) -> Merge/1
  Initial Condition/1 -> Bus Creator/4  "ISGOut_Load"
  "Initial Condition "/1 -> Bus Creator/6  "EngineOut_Load"
  Memory/1 -> Switch1/3
  Clutch Copy/1 -> Switch1/1
  Switch1/1 -> Memory/1, ClutchOut.Pos/1
  Switch/1 -> GearBoxOut.GearNoTrg/1
  GearNoTrg Copy/1 -> Switch/1
  NOTSET/1 -> Switch/3
  Logical Operator1/1 -> Switch/2
  Compare To Constant/1 -> Switch1/2, Logical Operator1/1
  Logical Operator/1 -> Logical Operator1/2
  Compare To Constant2/1 -> Logical Operator/2
  Compare To Constant1/1 -> Logical Operator/1
  Merge/1 -> Bus Selector/1
  OperState_Driving/1(Out) -> Merge/5
  OperState_PowerOn/1(Out) -> Merge/4
  OperState_PowerAccessory/1(Out) -> Merge/3
  OperState_PowerOff/1(Out) -> Merge/2
  Bus Selector1/5 -> "Initial Condition "/1  "<EngineOut_Load>"
  Bus Selector1/4 -> Bus Creator/5  "<EngineOut_set_ISC>"
  Bus Selector1/3 -> Initial Condition/1  "<ISGOut_Load>"
  Bus Selector1/2 -> Bus Creator/3  "<Ignition>"
  Bus Selector1/1 -> Bus Creator/2  "<OperationState>"
  Switch OperationState/1 -> OperState_Absent/Action
  Switch OperationState/5 -> OperState_Driving/Action
  Switch OperationState/4 -> OperState_PowerOn/Action
  Switch OperationState/2 -> OperState_PowerOff/Action
  Gas/1 -> OperState_Driving/3(Gas)
  GBKind/1 -> OperState_PowerOn/6(GBKind)
  SelectorCtrl/1 -> OperState_PowerOn/5(SelectorCtrl)
  Clutch/1 -> OperState_PowerOn/4(Clutch)
  Brake/1 -> OperState_PowerOn/3(Brake)
  GearNoTrg/1 -> OperState_PowerOn/2(GearNoTrg)
  Bus Selector/4 -> EngineOut.Load/1  "<EngineOut_Load>"
  Bus Selector/3 -> EngineOut.set_ISC/1  "<EngineOut_set_ISC>"
  Bus Selector/2 -> ISGOut.Load/1  "<ISGOut_Load>"
  Bus Creator/1 -> OperState_Driving/1(In), OperState_PowerOn/1(In), OperState_PowerAccessory/1(In), OperState_PowerOff/1(In), OperState_Absent/1(In)
  Key/1 -> Bus Creator/1
  Bus Selector2/1 -> Switch OperationState/1  "<OperationState>"
  last cycle/1 -> Bus Selector1/1, Bus Selector2/1  "last cycle"
  EngineIn.Engine_on/1 -> OperState_Driving/2(EngineIn.Engine_on), OperState_PowerOn/7(EngineIn_Engine_on)
  Bus Selector/5 -> Compare To Constant3/1, OperationState/1  "<OperationState>"
  Bus Selector/1 -> Ignition/1  "<Ignition>"
  Switch OperationState/3 -> OperState_PowerAccessory/Action
  Mode_EngineDrive/1 -> StrategyMode/1
  No_WarnError/1 -> OperationError/1

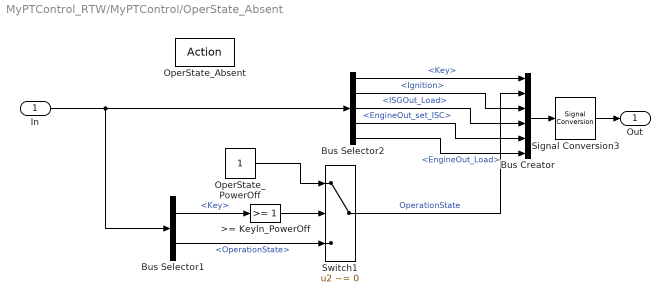
== system MyPTControl_RTW/MyPTControl/OperState_Absent ==
  In : Inport
  OperState_Absent : ActionPort
  >= KeyIn_PowerOff : simulink/Logic and Bit Operations/Compare To Constant  relop=>=  const=1  OutDataTypeStr=uint8  ZeroCross=off
  Bus Creator : BusCreator  Inputs=6
  Bus Selector1 : BusSelector  OutputSignals=Key,OperationState
  Bus Selector2 : BusSelector  OutputSignals=Key,Ignition,ISGOut_Load,EngineOut_set_ISC,EngineOut_Load
  OperState_PowerOff : Constant
  Signal Conversion3 : SignalConversion  ConversionOutput=Bus copy  OverrideOpt=off
  Switch1 : Switch  Criteria=u2 ~= 0  Threshold=1  SaturateOnIntegerOverflow=off  InputSameDT=off
  Out : Outport  VectorParamsAs1DForOutWhenUnconnected=off
  wires:
  >= KeyIn_PowerOff/1 -> Switch1/2
  Bus Selector2/5 -> Bus Creator/6  "<EngineOut_Load>"
  Bus Selector2/4 -> Bus Creator/5  "<EngineOut_set_ISC>"
  Bus Selector2/3 -> Bus Creator/4  "<ISGOut_Load>"
  Bus Selector2/2 -> Bus Creator/3  "<Ignition>"
  Bus Selector2/1 -> Bus Creator/1  "<Key>"
  Switch1/1 -> Bus Creator/2  "OperationState"
  Signal Conversion3/1 -> Out/1
  Bus Creator/1 -> Signal Conversion3/1
  Bus Selector1/2 -> Switch1/3  "<OperationState>"
  OperState_PowerOff/1 -> Switch1/1
  Bus Selector1/1 -> >= KeyIn_PowerOff/1  "<Key>"
  In/1 -> Bus Selector2/1, Bus Selector1/1

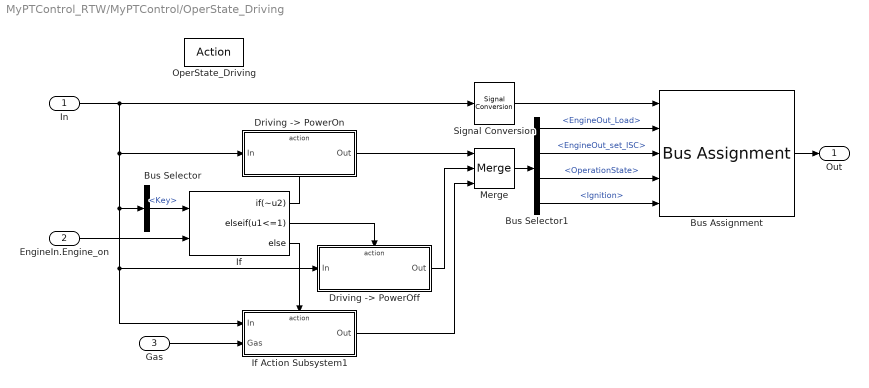
== system MyPTControl_RTW/MyPTControl/OperState_Driving ==
  In : Inport
  EngineIn.Engine_on : Inport  Port=2
  Gas : Inport  Port=3
  OperState_Driving : ActionPort
  Bus Assignment : BusAssignment  AssignedSignals=EngineOut_Load,EngineOut_set_ISC,OperationState,Ignition
  Bus Selector : BusSelector  OutputSignals=Key
  Bus Selector1 : BusSelector  OutputSignals=EngineOut_Load,EngineOut_set_ISC,OperationState,Ignition
  "Driving -> PowerOff" : Subsystem  TreatAsAtomicUnit=on
  "Driving -> PowerOn" : Subsystem  TreatAsAtomicUnit=on
  If : If  NumInputs=2  IfExpression=~u2  ElseIfExpressions=u1<=1
  If Action Subsystem1 : Subsystem  TreatAsAtomicUnit=on
  Merge : Merge  Inputs=3
  Signal Conversion : SignalConversion  ConversionOutput=Bus copy  OverrideOpt=off
  Out : Outport  VectorParamsAs1DForOutWhenUnconnected=off
  wires:
  Signal Conversion/1 -> Bus Assignment/1
  "Driving -> PowerOff"/1(Out) -> Merge/2
  Gas/1 -> If Action Subsystem1/2(Gas)
  Bus Selector1/4 -> Bus Assignment/5  "<Ignition>"
  Bus Selector1/3 -> Bus Assignment/4  "<OperationState>"
  Bus Selector1/2 -> Bus Assignment/3  "<EngineOut_set_ISC>"
  Bus Selector1/1 -> Bus Assignment/2  "<EngineOut_Load>"
  "Driving -> PowerOn"/1(Out) -> Merge/1
  If Action Subsystem1/1(Out) -> Merge/3
  EngineIn.Engine_on/1 -> If/2
  Bus Selector/1 -> If/1  "<Key>"
  If/2 -> "Driving -> PowerOff"/Action
  If/1 -> "Driving -> PowerOn"/Action
  If/3 -> If Action Subsystem1/Action
  In/1 -> Signal Conversion/1, If Action Subsystem1/1(In), "Driving -> PowerOff"/1(In), Bus Selector/1, "Driving -> PowerOn"/1(In)
  Bus Assignment/1 -> Out/1
  Merge/1 -> Bus Selector1/1

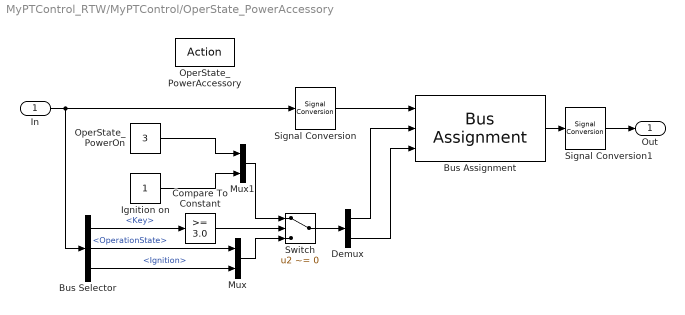
== system MyPTControl_RTW/MyPTControl/OperState_PowerAccessory ==
  In : Inport
  OperState_PowerAccessory : ActionPort
  Bus Assignment : BusAssignment  AssignedSignals=OperationState,Ignition
  Bus Selector : BusSelector  OutputSignals=Key,OperationState,Ignition
  Compare To Constant : simulink/Logic and Bit Operations/Compare To Constant  relop=>=  const=3.0  OutDataTypeStr=uint8  ZeroCross=off
  Demux : Demux  Outputs=2
  Ignition on : Constant
  Mux : Mux  Inputs=2
  Mux1 : Mux  Inputs=2
  OperState_PowerOn : Constant  Value=3
  Signal Conversion : SignalConversion  ConversionOutput=Bus copy  OverrideOpt=off
  Signal Conversion1 : SignalConversion  ConversionOutput=Bus copy  OverrideOpt=off
  Switch : Switch  Criteria=u2 ~= 0  Threshold=3  SaturateOnIntegerOverflow=off  InputSameDT=off
  Out : Outport  VectorParamsAs1DForOutWhenUnconnected=off
  wires:
  Compare To Constant/1 -> Switch/2
  Signal Conversion1/1 -> Out/1
  Signal Conversion/1 -> Bus Assignment/1
  OperState_PowerOn/1 -> Mux1/1
  In/1 -> Signal Conversion/1, Bus Selector/1
  Bus Assignment/1 -> Signal Conversion1/1
  Ignition on/1 -> Mux1/2
  Mux1/1 -> Switch/1
  Mux/1 -> Switch/3
  Bus Selector/3 -> Mux/2  "<Ignition>"
  Bus Selector/2 -> Mux/1  "<OperationState>"
  Demux/2 -> Bus Assignment/3
  Demux/1 -> Bus Assignment/2
  Switch/1 -> Demux/1
  Bus Selector/1 -> Compare To Constant/1  "<Key>"

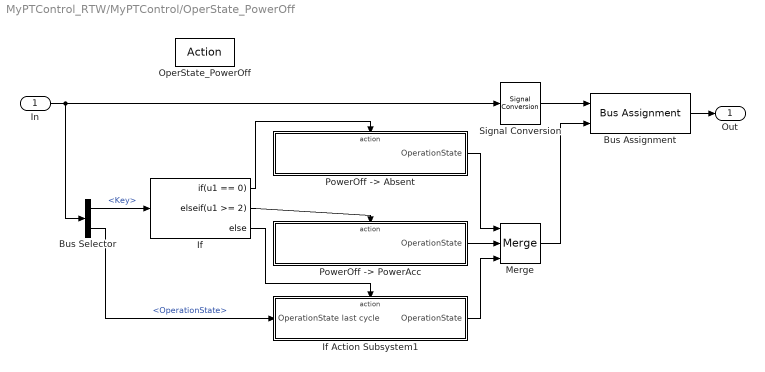
== system MyPTControl_RTW/MyPTControl/OperState_PowerOff ==
  In : Inport
  OperState_PowerOff : ActionPort
  Bus Assignment : BusAssignment  AssignedSignals=OperationState
  Bus Selector : BusSelector  OutputSignals=Key,OperationState
  If : If  IfExpression=u1 == 0  ElseIfExpressions=u1 >= 2
  If Action Subsystem1 : Subsystem  TreatAsAtomicUnit=on
  Merge : Merge  Inputs=3
  "PowerOff -> Absent" : Subsystem  TreatAsAtomicUnit=on
  "PowerOff -> PowerAcc" : Subsystem  TreatAsAtomicUnit=on
  Signal Conversion : SignalConversion  ConversionOutput=Bus copy  OverrideOpt=off
  Out : Outport  VectorParamsAs1DForOutWhenUnconnected=off
  wires:
  Signal Conversion/1 -> Bus Assignment/1
  Bus Selector/1 -> If/1  "<Key>"
  In/1 -> Signal Conversion/1, Bus Selector/1
  Bus Assignment/1 -> Out/1
  If/3 -> If Action Subsystem1/Action
  If Action Subsystem1/1(OperationState) -> Merge/3
  "PowerOff -> PowerAcc"/1(OperationState) -> Merge/2
  If/2 -> "PowerOff -> PowerAcc"/Action
  Bus Selector/2 -> If Action Subsystem1/1(OperationState last cycle)  "<OperationState>"
  "PowerOff -> Absent"/1(OperationState) -> Merge/1
  Merge/1 -> Bus Assignment/2
  If/1 -> "PowerOff -> Absent"/Action
